simulink model "simulink_testfile"  (R2013b)
settings: Solver=ode45  StartTime=0.0  StopTime=10.0  MaxStep=1e-3  RelTol=1e-3
values from neighbouring files (symbols this model uses):
  A = [0 1; -1/T^2 -2*xi/T]    [set_params_simulink_testfile.m]
  B = [0;V/T^2]    [set_params_simulink_testfile.m]
  D = 0    [set_params_simulink_testfile.m]
  G_tf = tf([V],[T^2 2*xi*T 1])    [set_params_simulink_testfile.m]
  T = 0.5    [set_params_simulink_testfile.m]
  Ta = 0.1    [set_params_simulink_testfile.m]    (also in set_params_test_matlabfunc.m = 0.01)
  V = 2    [set_params_simulink_testfile.m]
  xi = 0.2    [set_params_simulink_testfile.m]
libraries: cstblocks x2, simulink x1
settings Model: Creator=tk  LastModifiedBy=zp
settings DataIOCC: SignalLoggingSaveFormat=ModelDataLogs
settings OptimizationCC: ExpressionDepthLimit=2147483647  InitFltsAndDblsToZero=on
settings DebuggingCC: SaveWithParameterizedLinksMsg=none  FcnCallInpInsideContextMsg=UseLocalSettings  StateNameClashWarn=warning
settings GRTTargetCC: CombineOutputUpdateFcns=off  GRTInterface=on

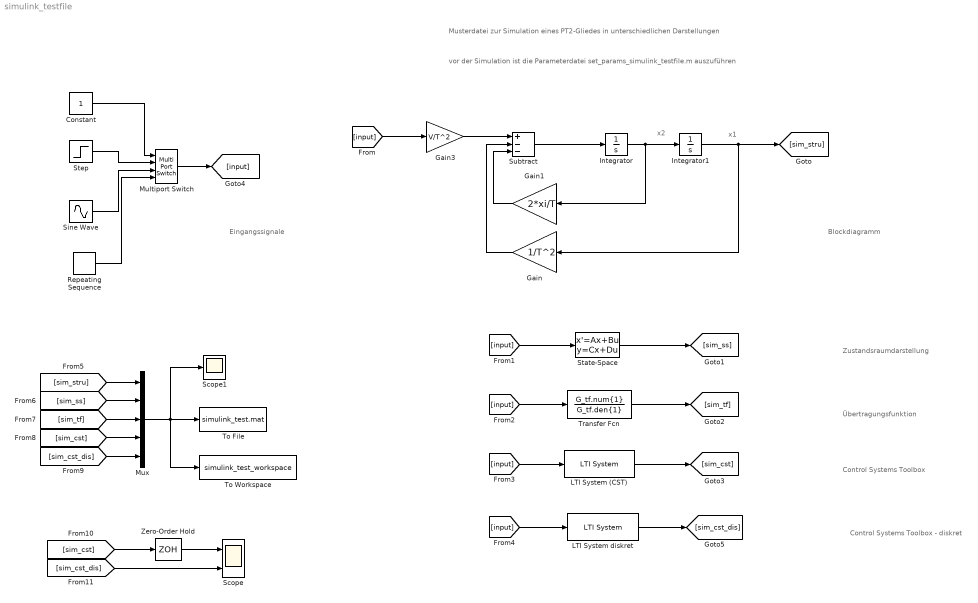
== system simulink_testfile ==
  note: x2
  note: x1
  note: Musterdatei zur Simulation eines PT2-Gliedes in unterschiedlichen Darstellungen
  note: Blockdiagramm
  note: Zustandsraumdarstellung
  note: Übertragungsfunktion
  note: Control Systems Toolbox
  note: Control Systems Toolbox - diskret
  note: vor der Simulation ist die Parameterdatei set_params_simulink_testfile.m auszuführen
  note: Eingangssignale
  Constant : Constant
  Gain : Gain  Gain=1/T^2
  Gain1 : Gain  Gain=2*xi/T
  Gain3 : Gain  Gain=V/T^2
  Integrator : Integrator
  Integrator1 : Integrator
  LTI System (CST) : cstblocks/LTI System  sys=sys  IC=[]
  LTI System diskret : cstblocks/LTI System  sys=G_z  IC=[]
  Multiport Switch : MultiPortSwitch
  Mux : Mux  Inputs=5
  Repeating Sequence : simulink/Sources/Repeating Sequence  rep_seq_t=[0 2]  rep_seq_y=[0 2]
  Scope : Scope  NumInputPorts=2
      settings: YMin=-5~-5  YMax=5~5
  Scope1 : Scope
  Sine Wave : Sin  SampleTime=0
  State-Space : StateSpace  A=A  B=B  C=C'  D=D  X0=0
  Step : Step  SampleTime=0
  Subtract : Sum  Inputs=+--
  To File : ToFile  Filename=simulink_test.mat
  To Workspace : ToWorkspace  VariableName=simulink_test_workspace  SampleTime=-1  SaveFormat=Structure With Time
  Transfer Fcn : TransferFcn  Numerator=G_tf.num{1}  Denominator=G_tf.den{1}
  Zero-Order Hold : ZeroOrderHold  SampleTime=Ta
  wires:
  Subtract/1 -> Integrator/1
  Integrator/1 -> Integrator1/1, Gain1/1
  Gain1/1 -> Subtract/3
  Gain/1 -> Subtract/2
  Integrator1/1 -> Gain/1, [sim_stru]
  Gain3/1 -> Subtract/1
  Constant/1 -> Multiport Switch/1
  Step/1 -> Multiport Switch/2
  Sine Wave/1 -> Multiport Switch/3
  Repeating Sequence/1 -> Multiport Switch/4
  Multiport Switch/1 -> [input]
  [input] -> Gain3/1
  [input] -> State-Space/1
  [input] -> Transfer Fcn/1
  [input] -> LTI System (CST)/1
  State-Space/1 -> [sim_ss]
  Transfer Fcn/1 -> [sim_tf]
  LTI System (CST)/1 -> [sim_cst]
  [input] -> LTI System diskret/1
  LTI System diskret/1 -> [sim_cst_dis]
  [sim_stru] -> Mux/1
  [sim_ss] -> Mux/2
  [sim_tf] -> Mux/3
  [sim_cst] -> Mux/4
  [sim_cst_dis] -> Mux/5
  Mux/1 -> To File/1, To Workspace/1, Scope1/1
  [sim_cst] -> Zero-Order Hold/1
  [sim_cst_dis] -> Scope/2
  Zero-Order Hold/1 -> Scope/1
